simulink model "IndustrialMicrogrid"  (R2023a)
settings: Solver=FixedStepDiscrete  StartTime=0.0  StopTime=10  FixedStep=Ts  RelTol=1e-3
PostLoadFcn:
  | IndustrialMicrogridInputData
  | GfmGridFormingConverterInputParameters
model workspace (MAT data in the model file):
  caseNum = 2
undefined symbols (not defined in the file): base, BESS, DiscIntNeverNeededParam, grid, Grid, gridInverter, machine, microgrid, PV, PVInverter, PVTransformer, scrFactorRg, scrFactorXg, transformer, Ts
libraries: ee_lib x112, eeGeneralControl x104, nesl_utility_internal x64, simulink x56, nesl_utility x37, fl_lib x29, slpidlib x13, eeTransforms x11, eeTotalHarmonicDistorsion x8, eeRmsMeasurement x4, eeSinusoidalMeasurement x4, simulink_extras x2
(part 13 of 14)

== system IndustrialMicrogrid/MG1 Primary Substation/BESS and Controller/BESS/Grid-Forming Converter Control/Current Limiting/CurrentLimitingMethod/currentSaturation/If Action Subsystem ==
  Is : Inport
  Isd : Inport  Port=2
  Isq : Inport  Port=3
  Action Port : ActionPort
  Constant : Constant  Value=maxSatCurrentLimit
  Divide : Product  Inputs=*/
  Product : Product
  Product1 : Product
  Idmax : Outport
  Iqmax : Outport  Port=2
  wires:
  Constant/1 -> Divide/1
  Is/1 -> Divide/2
  Divide/1 -> Product1/2, Product/1
  Isd/1 -> Product1/1
  Isq/1 -> Product/2
  Product1/1 -> Idmax/1
  Product/1 -> Iqmax/1

== system IndustrialMicrogrid/MG1 Primary Substation/BESS and Controller/BESS/Grid-Forming Converter Control/Current Limiting/CurrentLimitingMethod/currentSaturation/If Action Subsystem1 ==
  Action Port : ActionPort
  Constant3 : Constant  Value=0
  Constant4 : Constant  Value=0
  Idmax : Outport
  Iqmax : Outport  Port=2
  wires:
  Constant4/1 -> Iqmax/1
  Constant3/1 -> Idmax/1

== system IndustrialMicrogrid/MG1 Primary Substation/BESS and Controller/BESS/Grid-Forming Converter Control/Grid Voltage Reactive Power Support/Modifying Reactive Power Reference/Changing the Power Reference/ActivePowerReference ==
  note: Ensure Pref sign is maintained
  Id : Inport
  Vd : Inport  Port=2
  Pref : Inport  Port=3
  Abs1 : Abs  SaturateOnIntegerOverflow=off
  Abs2 : Abs  SaturateOnIntegerOverflow=off
  Min : MinMax  Inputs=2
  Product : Product
  Product2 : Product
  Saturation : Saturate  UpperLimit=1  LowerLimit=-1
  Sign : Signum
  PrefNew : Outport
  wires:
  Pref/1 -> Abs1/1, Sign/1
  Id/1 -> Product/1
  Sign/1 -> Product2/2
  Abs1/1 -> Min/2
  Product/1 -> Abs2/1
  Min/1 -> Product2/1
  Product2/1 -> Saturation/1
  Abs2/1 -> Min/1
  Vd/1 -> Product/2
  Saturation/1 -> PrefNew/1

== system IndustrialMicrogrid/MG1 Primary Substation/BESS and Controller/BESS/Grid-Forming Converter Control/Grid Voltage Reactive Power Support/Modifying Reactive Power Reference/Changing the Power Reference/EstimateIdForGivenIq ==
  Iq : Inport
  Add Constant1 : Bias  Bias=1*1  SaturateOnIntegerOverflow=off
  Gain : Gain  Gain=-1
  Gain3 : Gain  Gain=0.9
  Sqrt : Sqrt
  Square : Math  Operator=square
  Id : Outport
  wires:
  Square/1 -> Gain/1
  Gain3/1 -> Id/1
  Gain/1 -> Add Constant1/1
  Sqrt/1 -> Gain3/1
  Add Constant1/1 -> Sqrt/1
  Iq/1 -> Square/1

== system IndustrialMicrogrid/MG1 Primary Substation/BESS and Controller/BESS/Grid-Forming Converter Control/Grid Voltage Reactive Power Support/Modifying Reactive Power Reference/Changing the Power Reference/EstimateIqForReactivePower ==
  note: Computing minimum reactive power as per GC0137
  Vmin : Inport
  Vd : Inport  Port=2
  Vs : Inport  Port=3
  Abs : Abs  SaturateOnIntegerOverflow=off
  Add : Sum
  Add Constant : Bias  Bias=1  SaturateOnIntegerOverflow=off
  GC0137 line slope : Gain  Gain=-1.4578
  Gain4 : Gain  Gain=1.5
  Saturation : Saturate  UpperLimit=1  LowerLimit=0
  Saturation1 : Saturate  UpperLimit=1  LowerLimit=-1
  Subtract : Sum  Inputs=+-
  Iq : Outport
  wires:
  Abs/1 -> GC0137 line slope/1
  GC0137 line slope/1 -> Add Constant/1
  Subtract/1 -> Gain4/1
  Saturation1/1 -> Add/1
  Gain4/1 -> Saturation1/1
  Vmin/1 -> Subtract/1
  Vs/1 -> Abs/1
  Vd/1 -> Subtract/2
  Add/1 -> Saturation/1
  Saturation/1 -> Iq/1
  Add Constant/1 -> Add/2

== system IndustrialMicrogrid/MG1 Primary Substation/BESS and Controller/BESS/Grid-Forming Converter Control/Grid Voltage Reactive Power Support/Modifying Reactive Power Reference/Changing the Power Reference/ReactivePowerReference ==
  Vd : Inport
  Iq : Inport  Port=2
  Compute Power : Product
  Constant : Constant  Value=0.3
  Gain2 : Gain  Gain=1.05
  Switch : Switch  Criteria=u2 > Threshold  Threshold=0.3  SaturateOnIntegerOverflow=off  InputSameDT=off
  QrefNew : Outport
  wires:
  Compute Power/1 -> QrefNew/1
  Gain2/1 -> Compute Power/2
  Constant/1 -> Switch/3
  Iq/1 -> Gain2/1
  Vd/1 -> Switch/2, Switch/1
  Switch/1 -> Compute Power/1

== system IndustrialMicrogrid/MG1 Primary Substation/BESS and Controller/BESS/Grid-Forming Converter Control/Measurement/Frequency Measurement/Frequency Measurement/If Action Subsystem ==
  V : Inport
  Time : Inport  Port=2
  Action Port : ActionPort  ActionPortLabel=if(u1 > 0.9)
  Constant1 : Constant  Value=initialFrequency
  Delay : Delay  DelayLength=1
  Delay1 : Delay  DelayLength=1
  Frequency estimation : Subsystem  TreatAsAtomicUnit=on
  Hit Crossing : HitCross
  Second-Order Filter : eeGeneralControl/Second-Order Filter  Commented=through  FilterType=Low-pass  fn=initialFrequency  Zeta=1  Ts=sampleTime  A0=0  Ph0=0  f0=0  b0=0
      settings: LibrarySourceBlock=ee_sl_lib/General Control/Second-Order Filter
  Switch : Switch  Criteria=u2 > Threshold  Threshold=1  SaturateOnIntegerOverflow=off  InputSameDT=off
  Freq : Outport
  wires:
  Second-Order Filter/1 -> Delay/1, Frequency estimation/1(sk), Hit Crossing/1
  Delay1/1 -> Frequency estimation/4(k-1)
  Hit Crossing/1 -> Frequency estimation/Trigger
  Delay/1 -> Frequency estimation/2(sk-1)
  V/1 -> Second-Order Filter/1
  Time/1 -> Switch/2, Delay1/1, Frequency estimation/3(k)
  Frequency estimation/1(f) -> Switch/1
  Constant1/1 -> Switch/3
  Switch/1 -> Freq/1

== system IndustrialMicrogrid/MG1 Primary Substation/BESS and Controller/BESS/Grid-Forming Converter Control/Measurement/Frequency Measurement/Frequency Measurement/If Action Subsystem1 ==
  Action Port : ActionPort  ActionPortLabel=else
  Constant1 : Constant  Value=initialFrequency
  Out1 : Outport
  wires:
  Constant1/1 -> Out1/1

== system IndustrialMicrogrid/MG1 Primary Substation/BESS and Controller/BESS/Grid-Forming Converter Control/Measurement/Frequency Measurement/Frequency Measurement/Postive Sequence ==
  abc : Inport
  Complex to Real-Imag : ComplexToRealImag
  Demux : Demux  Outputs=3
  Symmetrical-Components Transform : eeTransforms/Symmetrical-Components Transform  PowerInvariant=off
      settings: LibrarySourceBlock=|
      | ee_sl_lib/Mathematical
      | Transforms/Symmetrical-Components
      | Transform
  Terminator : Terminator
  Terminator1 : Terminator
  Terminator2 : Terminator
  Transpose : Math  Operator=transpose
  posSeq : Outport
  wires:
  Transpose/1 -> Symmetrical-Components Transform/1
  Symmetrical-Components Transform/1 -> Demux/1
  Complex to Real-Imag/1 -> posSeq/1
  Demux/1 -> Complex to Real-Imag/1
  abc/1 -> Transpose/1
  Complex to Real-Imag/2 -> Terminator/1
  Demux/2 -> Terminator1/1
  Demux/3 -> Terminator2/1

== system IndustrialMicrogrid/MG1 Primary Substation/BESS and Controller/BESS/Grid-Forming Converter Control/Power Control/ActivePowerControl/vsmControl/Damping Frequency ==
  fref : Inport
  ConstantFreqReference : Subsystem  VariantControl=constFreq
  WithFrequencyMeasurement : Subsystem  VariantControl=freqMeas
  fmeas : Outport

== system IndustrialMicrogrid/MG1 Primary Substation/BESS and Controller/BESS/Grid-Forming Converter Control/Power Control/ActivePowerControl/vsmControl/Power Reference Selection ==
  cntrlflag : Inport
  Pref : Inport  Port=2
  fref : Inport  Port=3
  Wsm : Inport  Port=4
  If : If
  If Action Subsystem : Subsystem  TreatAsAtomicUnit=on
  If Action Subsystem1 : Subsystem  TreatAsAtomicUnit=on
  Merge : Merge
  power : Outport
  wires:
  If Action Subsystem1/1(Power) -> Merge/2
  If/1 -> If Action Subsystem/Action
  Pref/1 -> If Action Subsystem/1(Pref)
  [Wsm] -> If Action Subsystem1/2(Wsm)
  fref/1 -> If Action Subsystem1/1(fref)
  [Wsm] -> If Action Subsystem/2(Wsm)
  If Action Subsystem/1(Power) -> Merge/1
  If/2 -> If Action Subsystem1/Action
  cntrlflag/1 -> If/1
  Merge/1 -> power/1
  Wsm/1 -> [Wsm]

== system IndustrialMicrogrid/MG1 Primary Substation/BESS and Controller/BESS/Grid-Forming Converter Control/Power Control/ReactiveControl/Voltage  Reference Selection/If Action Subsystem ==
  note: Vs-delV
  Qref : Inport
  Qmeas : Inport  Port=2
  Action Port : ActionPort  ActionPortLabel=if(u1 > 0)
  Constant : Constant  Value=voltreference
  Gain : Gain  Gain=QVoltDroop
  Low-Pass Filter (Discrete or Continuous) : eeGeneralControl/Low-Pass Filter (Discrete or Continuous)  K=1  T=QVoltFilterTC  B=inf  A=-inf  init_option=Specify as parameter  x0=0  Ts=activePowerSampleTime
  Product1 : Product
  Sum : Sum  Inputs=|+-
  Sum1 : Sum  Inputs=|++
  Vd : Outport
  wires:
  Constant/1 -> Product1/2, Sum1/2
  Qmeas/1 -> Low-Pass Filter (Discrete or Continuous)/1
  Gain/1 -> Sum1/1
  Qref/1 -> Sum/1
  Low-Pass Filter (Discrete or Continuous)/1 -> Sum/2
  Sum/1 -> Gain/1
  Sum1/1 -> Product1/1
  Product1/1 -> Vd/1  "V"

== system IndustrialMicrogrid/MG1 Primary Substation/BESS and Controller/BESS/Grid-Forming Converter Control/Power Control/ReactiveControl/Voltage  Reference Selection/If Action Subsystem1 ==
  note: Vs-delV
  Vref : Inport
  Vmeas : Inport  Port=2
  Action Port : ActionPort  ActionPortLabel=else
  Constant : Constant  Value=voltreference
  Gain : Gain  Gain=1/QVoltDroop
  Low-Pass Filter (Discrete or Continuous) : eeGeneralControl/Low-Pass Filter (Discrete or Continuous)  K=1  T=QVoltFilterTC  B=inf  A=-inf  init_option=Specify as parameter  x0=0  Ts=activePowerSampleTime
  Product1 : Product
  Scope : Scope
  Scope1 : Scope
  Scope2 : Scope
  Sum : Sum  Inputs=|+-
  Sum1 : Sum  Inputs=|++
  Voltage : Outport
  wires:
  Vref/1 -> Voltage/1, Product1/1, Sum/1
  Gain/1 -> Sum1/1
  Vmeas/1 -> Low-Pass Filter (Discrete or Continuous)/1
  Constant/1 -> Sum1/2
  Low-Pass Filter (Discrete or Continuous)/1 -> Sum/2, Scope1/1
  Sum/1 -> Scope2/1, Gain/1
  Product1/1 -> Scope/1  "V"
  Sum1/1 -> Product1/2

== system IndustrialMicrogrid/MG2 Primary Substation/BESS and Controller 2/BESS/Grid-Forming Converter Control/Current Limiting/CurrentLimitingMethod/currentLimitAndVirtual/Current Saturation ==
  note: Vs-delV
  Id : Inport
  Iq : Inport  Port=2
  Imaxsat : Inport  Port=3
  Enable : EnablePort
  Compare : Subsystem
  Constant1 : Constant  Value=0
  Constant2 : Constant  Value=0
  If : If
  If Action Subsystem : Subsystem  TreatAsAtomicUnit=on
  If Action Subsystem1 : Subsystem  TreatAsAtomicUnit=on
  Math Function : Math  Operator=hypot
  Merge : Merge
  Merge1 : Merge
  Subtract : Sum  Inputs=+-
  delVd : Outport
  delVq : Outport  Port=2
  idmax : Outport  Port=3
  iqmax : Outport  Port=4
  wires:
  Iq/1 -> [Isq], Math Function/2
  If/1 -> If Action Subsystem/Action
  If Action Subsystem1/1(Idmax) -> Merge/2
  Constant2/1 -> delVq/1
  Math Function/1 -> [Is], Subtract/2
  If/2 -> If Action Subsystem1/Action
  If Action Subsystem/2(Iqmax) -> Merge1/1
  Subtract/1 -> Compare/1(u)
  Compare/1(Out1) -> If/1
  If Action Subsystem/1(Idmax) -> Merge/1
  [Is] -> If Action Subsystem/1(Is)
  Id/1 -> [Isd], Math Function/1
  If Action Subsystem1/2(Iqmax) -> Merge1/2
  Merge/1 -> idmax/1
  [Isd] -> If Action Subsystem/2(Isd)
  Constant1/1 -> delVd/1
  [Isq] -> If Action Subsystem/3(Isq)
  Merge1/1 -> iqmax/1
  Imaxsat/1 -> [Imax], Subtract/1
  [Imax] -> If Action Subsystem/4(maxI)

== system IndustrialMicrogrid/MG2 Primary Substation/BESS and Controller 2/BESS/Grid-Forming Converter Control/Current Limiting/CurrentLimitingMethod/currentLimitAndVirtual/No Fault Ride Through ==
  Id : Inport
  Iq : Inport  Port=2
  Enable : EnablePort
  Constant{1..4} (4 alike) : Constant  Value=0
  Terminator : Terminator
  Terminator1 : Terminator
  delVd : Outport
  delVq : Outport  Port=2
  idmax : Outport  Port=3
  iqmax : Outport  Port=4
  wires:
  Constant3/1 -> iqmax/1
  Constant2/1 -> idmax/1
  Constant1/1 -> delVd/1
  Constant4/1 -> delVq/1
  Id/1 -> Terminator/1
  Iq/1 -> Terminator1/1

== system IndustrialMicrogrid/MG2 Primary Substation/BESS and Controller 2/BESS/Grid-Forming Converter Control/Current Limiting/CurrentLimitingMethod/currentLimitAndVirtual/VI ==
  note: Resistance coefficient
  note: X/R ratio
  Id : Inport
  Iq : Inport  Port=2
  Imax : Inport  Port=3
  Enable : EnablePort
  Constant1 : Constant  Value=0
  Constant2 : Constant  Value=0
  Constant3 : Constant  Value=0
  Gain : Gain  Gain=ctLimitVirtualImp
  Gain1 : Gain  Gain=ctLimitXbyR
  Low-Pass Filter : eeGeneralControl/Low-Pass Filter (Discrete or Continuous)  K=1  T=currentVITimeConst  B=inf  A=-inf  init_option=Inherited from block input  x0=0  Ts=-1
  Math Function : Math  Operator=hypot
  Product{,1..3} (4 alike) : Product
  Relay1 : Relay  OnSwitchValue=0.01  OffSwitchValue=-0.1
  Saturation : Saturate  UpperLimit=1  LowerLimit=-1
  Saturation1 : Saturate  UpperLimit=1  LowerLimit=-1
  Sum : Sum  Inputs=|+-
  Sum1 : Sum  Inputs=|+-
  Sum2 : Sum  Inputs=++|
  Switch : Switch  Criteria=u2 > Threshold  SaturateOnIntegerOverflow=off  InputSameDT=off
  delVd : Outport
  delVq : Outport  Port=2
  idmax : Outport  Port=3
  iqmax : Outport  Port=4
  wires:
  Gain1/1 -> Product1/2, Product2/1
  Product3/1 -> Sum2/2
  Id/1 -> Math Function/1, [Igd]
  Sum2/1 -> Saturation1/1
  Sum/1 -> Gain/1, Relay1/1
  Sum1/1 -> Saturation/1
  Product/1 -> Sum1/1
  [Igq] -> Product3/1, Product2/2
  Iq/1 -> [Igq], Math Function/2
  Math Function/1 -> Low-Pass Filter/1  "Is"
  Switch/1 -> Product3/2, Product/1, Gain1/1
  [Igd] -> Product1/1, Product/2
  Saturation1/1 -> delVq/1
  Product1/1 -> Sum2/1
  Product2/1 -> Sum1/2
  Gain/1 -> Switch/1
  Constant1/1 -> Switch/3
  Saturation/1 -> delVd/1
  Constant3/1 -> iqmax/1
  Constant2/1 -> idmax/1
  Relay1/1 -> Switch/2
  Low-Pass Filter/1 -> Sum/1
  Imax/1 -> Sum/2  "IsMaximum"

== system IndustrialMicrogrid/MG2 Primary Substation/BESS and Controller 2/BESS/Grid-Forming Converter Control/Current Limiting/CurrentLimitingMethod/currentSaturation/Compare ==
  u : Inport
  AND : Logic  IconShape=distinctive  AllPortsSameDT=off  OutDataTypeStr=boolean
  Compare To Constant : simulink/Logic and Bit Operations/Compare To Constant  relop=>  const=ctLimitDelayTime  OutDataTypeStr=boolean
  Compare To Zero : simulink/Logic and Bit Operations/Compare To Zero  relop=<=  OutDataTypeStr=boolean
  Data Type Conversion : DataTypeConversion  SaturateOnIntegerOverflow=off  RndMeth=Floor
  Data Type Conversion1 : DataTypeConversion  SaturateOnIntegerOverflow=off  RndMeth=Floor
  Discrete-Time Integrator : DiscreteIntegrator  IntegratorMethod=Integration: Backward Euler  ExternalReset=level  SampleTime=currentControlTs  LimitOutput=on  UpperSaturationLimit=ctLimitDelayTime*2  LowerSaturationLimit=0  ICPrevOutput=DiscIntNeverNeededParam  ICPrevScaledInput=DiscIntNeverNeededParam
  Out1 : Outport
  wires:
  AND/1 -> Data Type Conversion/1
  Compare To Zero/1 -> Data Type Conversion1/1
  Compare To Constant/1 -> AND/2
  u/1 -> Compare To Zero/1
  Discrete-Time Integrator/1 -> Compare To Constant/1
  Data Type Conversion/1 -> Out1/1
  Data Type Conversion1/1 -> Discrete-Time Integrator/2, Discrete-Time Integrator/1, AND/1

== system IndustrialMicrogrid/MG2 Primary Substation/BESS and Controller 2/BESS/Grid-Forming Converter Control/Current Limiting/CurrentLimitingMethod/currentSaturation/If Action Subsystem ==
  Is : Inport
  Isd : Inport  Port=2
  Isq : Inport  Port=3
  Action Port : ActionPort
  Constant : Constant  Value=maxSatCurrentLimit
  Divide : Product  Inputs=*/
  Product : Product
  Product1 : Product
  Idmax : Outport
  Iqmax : Outport  Port=2
  wires:
  Constant/1 -> Divide/1
  Is/1 -> Divide/2
  Divide/1 -> Product1/2, Product/1
  Isd/1 -> Product1/1
  Isq/1 -> Product/2
  Product1/1 -> Idmax/1
  Product/1 -> Iqmax/1

== system IndustrialMicrogrid/MG2 Primary Substation/BESS and Controller 2/BESS/Grid-Forming Converter Control/Current Limiting/CurrentLimitingMethod/currentSaturation/If Action Subsystem1 ==
  Action Port : ActionPort
  Constant3 : Constant  Value=0
  Constant4 : Constant  Value=0
  Idmax : Outport
  Iqmax : Outport  Port=2
  wires:
  Constant4/1 -> Iqmax/1
  Constant3/1 -> Idmax/1

== system IndustrialMicrogrid/MG2 Primary Substation/BESS and Controller 2/BESS/Grid-Forming Converter Control/Grid Voltage Reactive Power Support/Modifying Reactive Power Reference/Changing the Power Reference/ActivePowerReference ==
  note: Ensure Pref sign is maintained
  Id : Inport
  Vd : Inport  Port=2
  Pref : Inport  Port=3
  Abs1 : Abs  SaturateOnIntegerOverflow=off
  Abs2 : Abs  SaturateOnIntegerOverflow=off
  Min : MinMax  Inputs=2
  Product : Product
  Product2 : Product
  Saturation : Saturate  UpperLimit=1  LowerLimit=-1
  Sign : Signum
  PrefNew : Outport
  wires:
  Pref/1 -> Abs1/1, Sign/1
  Id/1 -> Product/1
  Sign/1 -> Product2/2
  Abs1/1 -> Min/2
  Product/1 -> Abs2/1
  Min/1 -> Product2/1
  Product2/1 -> Saturation/1
  Abs2/1 -> Min/1
  Vd/1 -> Product/2
  Saturation/1 -> PrefNew/1

== system IndustrialMicrogrid/MG2 Primary Substation/BESS and Controller 2/BESS/Grid-Forming Converter Control/Grid Voltage Reactive Power Support/Modifying Reactive Power Reference/Changing the Power Reference/EstimateIdForGivenIq ==
  Iq : Inport
  Add Constant1 : Bias  Bias=1*1  SaturateOnIntegerOverflow=off
  Gain : Gain  Gain=-1
  Gain3 : Gain  Gain=0.9
  Sqrt : Sqrt
  Square : Math  Operator=square
  Id : Outport
  wires:
  Square/1 -> Gain/1
  Gain3/1 -> Id/1
  Gain/1 -> Add Constant1/1
  Sqrt/1 -> Gain3/1
  Add Constant1/1 -> Sqrt/1
  Iq/1 -> Square/1

== system IndustrialMicrogrid/MG2 Primary Substation/BESS and Controller 2/BESS/Grid-Forming Converter Control/Grid Voltage Reactive Power Support/Modifying Reactive Power Reference/Changing the Power Reference/EstimateIqForReactivePower ==
  note: Computing minimum reactive power as per GC0137
  Vmin : Inport
  Vd : Inport  Port=2
  Vs : Inport  Port=3
  Abs : Abs  SaturateOnIntegerOverflow=off
  Add : Sum
  Add Constant : Bias  Bias=1  SaturateOnIntegerOverflow=off
  GC0137 line slope : Gain  Gain=-1.4578
  Gain4 : Gain  Gain=1.5
  Saturation : Saturate  UpperLimit=1  LowerLimit=0
  Saturation1 : Saturate  UpperLimit=1  LowerLimit=-1
  Subtract : Sum  Inputs=+-
  Iq : Outport
  wires:
  Abs/1 -> GC0137 line slope/1
  GC0137 line slope/1 -> Add Constant/1
  Subtract/1 -> Gain4/1
  Saturation1/1 -> Add/1
  Gain4/1 -> Saturation1/1
  Vmin/1 -> Subtract/1
  Vs/1 -> Abs/1
  Vd/1 -> Subtract/2
  Add/1 -> Saturation/1
  Saturation/1 -> Iq/1
  Add Constant/1 -> Add/2

== system IndustrialMicrogrid/MG2 Primary Substation/BESS and Controller 2/BESS/Grid-Forming Converter Control/Grid Voltage Reactive Power Support/Modifying Reactive Power Reference/Changing the Power Reference/ReactivePowerReference ==
  Vd : Inport
  Iq : Inport  Port=2
  Compute Power : Product
  Constant : Constant  Value=0.3
  Gain2 : Gain  Gain=1.05
  Switch : Switch  Criteria=u2 > Threshold  Threshold=0.3  SaturateOnIntegerOverflow=off  InputSameDT=off
  QrefNew : Outport
  wires:
  Compute Power/1 -> QrefNew/1
  Gain2/1 -> Compute Power/2
  Constant/1 -> Switch/3
  Iq/1 -> Gain2/1
  Vd/1 -> Switch/2, Switch/1
  Switch/1 -> Compute Power/1

== system IndustrialMicrogrid/MG2 Primary Substation/BESS and Controller 2/BESS/Grid-Forming Converter Control/Measurement/Frequency Measurement/Frequency Measurement/If Action Subsystem ==
  V : Inport
  Time : Inport  Port=2
  Action Port : ActionPort  ActionPortLabel=if(u1 > 0.9)
  Constant1 : Constant  Value=initialFrequency
  Delay : Delay  DelayLength=1
  Delay1 : Delay  DelayLength=1
  Frequency estimation : Subsystem  TreatAsAtomicUnit=on
  Hit Crossing : HitCross
  Second-Order Filter : eeGeneralControl/Second-Order Filter  Commented=through  FilterType=Low-pass  fn=initialFrequency  Zeta=1  Ts=sampleTime  A0=0  Ph0=0  f0=0  b0=0
      settings: LibrarySourceBlock=ee_sl_lib/General Control/Second-Order Filter
  Switch : Switch  Criteria=u2 > Threshold  Threshold=1  SaturateOnIntegerOverflow=off  InputSameDT=off
  Freq : Outport
  wires:
  Second-Order Filter/1 -> Delay/1, Frequency estimation/1(sk), Hit Crossing/1
  Delay1/1 -> Frequency estimation/4(k-1)
  Hit Crossing/1 -> Frequency estimation/Trigger
  Delay/1 -> Frequency estimation/2(sk-1)
  V/1 -> Second-Order Filter/1
  Time/1 -> Switch/2, Delay1/1, Frequency estimation/3(k)
  Frequency estimation/1(f) -> Switch/1
  Constant1/1 -> Switch/3
  Switch/1 -> Freq/1

== system IndustrialMicrogrid/MG2 Primary Substation/BESS and Controller 2/BESS/Grid-Forming Converter Control/Measurement/Frequency Measurement/Frequency Measurement/If Action Subsystem1 ==
  Action Port : ActionPort  ActionPortLabel=else
  Constant1 : Constant  Value=initialFrequency
  Out1 : Outport
  wires:
  Constant1/1 -> Out1/1

== system IndustrialMicrogrid/MG2 Primary Substation/BESS and Controller 2/BESS/Grid-Forming Converter Control/Measurement/Frequency Measurement/Frequency Measurement/Postive Sequence ==
  abc : Inport
  Complex to Real-Imag : ComplexToRealImag
  Demux : Demux  Outputs=3
  Symmetrical-Components Transform : eeTransforms/Symmetrical-Components Transform  PowerInvariant=off
      settings: LibrarySourceBlock=|
      | ee_sl_lib/Mathematical
      | Transforms/Symmetrical-Components
      | Transform
  Terminator : Terminator
  Terminator1 : Terminator
  Terminator2 : Terminator
  Transpose : Math  Operator=transpose
  posSeq : Outport
  wires:
  Transpose/1 -> Symmetrical-Components Transform/1
  Symmetrical-Components Transform/1 -> Demux/1
  Complex to Real-Imag/1 -> posSeq/1
  Demux/1 -> Complex to Real-Imag/1
  abc/1 -> Transpose/1
  Complex to Real-Imag/2 -> Terminator/1
  Demux/2 -> Terminator1/1
  Demux/3 -> Terminator2/1

== system IndustrialMicrogrid/MG2 Primary Substation/BESS and Controller 2/BESS/Grid-Forming Converter Control/Power Control/ActivePowerControl/vsmControl/Damping Frequency ==
  fref : Inport
  ConstantFreqReference : Subsystem  VariantControl=constFreq
  WithFrequencyMeasurement : Subsystem  VariantControl=freqMeas
  fmeas : Outport

== system IndustrialMicrogrid/MG2 Primary Substation/BESS and Controller 2/BESS/Grid-Forming Converter Control/Power Control/ActivePowerControl/vsmControl/Power Reference Selection ==
  cntrlflag : Inport
  Pref : Inport  Port=2
  fref : Inport  Port=3
  Wsm : Inport  Port=4
  If : If
  If Action Subsystem : Subsystem  TreatAsAtomicUnit=on
  If Action Subsystem1 : Subsystem  TreatAsAtomicUnit=on
  Merge : Merge
  power : Outport
  wires:
  If Action Subsystem1/1(Power) -> Merge/2
  If/1 -> If Action Subsystem/Action
  Pref/1 -> If Action Subsystem/1(Pref)
  [Wsm] -> If Action Subsystem1/2(Wsm)
  fref/1 -> If Action Subsystem1/1(fref)
  [Wsm] -> If Action Subsystem/2(Wsm)
  If Action Subsystem/1(Power) -> Merge/1
  If/2 -> If Action Subsystem1/Action
  cntrlflag/1 -> If/1
  Merge/1 -> power/1
  Wsm/1 -> [Wsm]

== system IndustrialMicrogrid/MG2 Primary Substation/BESS and Controller 2/BESS/Grid-Forming Converter Control/Power Control/ReactiveControl/Voltage  Reference Selection/If Action Subsystem ==
  note: Vs-delV
  Qref : Inport
  Qmeas : Inport  Port=2
  Action Port : ActionPort  ActionPortLabel=if(u1 > 0)
  Constant : Constant  Value=voltreference
  Gain : Gain  Gain=QVoltDroop
  Low-Pass Filter (Discrete or Continuous) : eeGeneralControl/Low-Pass Filter (Discrete or Continuous)  K=1  T=QVoltFilterTC  B=inf  A=-inf  init_option=Specify as parameter  x0=0  Ts=activePowerSampleTime
  Product1 : Product
  Sum : Sum  Inputs=|+-
  Sum1 : Sum  Inputs=|++
  Vd : Outport
  wires:
  Constant/1 -> Product1/2, Sum1/2
  Qmeas/1 -> Low-Pass Filter (Discrete or Continuous)/1
  Gain/1 -> Sum1/1
  Qref/1 -> Sum/1
  Low-Pass Filter (Discrete or Continuous)/1 -> Sum/2
  Sum/1 -> Gain/1
  Sum1/1 -> Product1/1
  Product1/1 -> Vd/1  "V"

== system IndustrialMicrogrid/MG2 Primary Substation/BESS and Controller 2/BESS/Grid-Forming Converter Control/Power Control/ReactiveControl/Voltage  Reference Selection/If Action Subsystem1 ==
  note: Vs-delV
  Vref : Inport
  Vmeas : Inport  Port=2
  Action Port : ActionPort  ActionPortLabel=else
  Constant : Constant  Value=voltreference
  Gain : Gain  Gain=1/QVoltDroop
  Low-Pass Filter (Discrete or Continuous) : eeGeneralControl/Low-Pass Filter (Discrete or Continuous)  K=1  T=QVoltFilterTC  B=inf  A=-inf  init_option=Specify as parameter  x0=0  Ts=activePowerSampleTime
  Product1 : Product
  Scope : Scope
  Scope1 : Scope
  Scope2 : Scope
  Sum : Sum  Inputs=|+-
  Sum1 : Sum  Inputs=|++
  Voltage : Outport
  wires:
  Vref/1 -> Voltage/1, Product1/1, Sum/1
  Gain/1 -> Sum1/1
  Vmeas/1 -> Low-Pass Filter (Discrete or Continuous)/1
  Constant/1 -> Sum1/2
  Low-Pass Filter (Discrete or Continuous)/1 -> Sum/2, Scope1/1
  Sum/1 -> Scope2/1, Gain/1
  Product1/1 -> Scope/1  "V"
  Sum1/1 -> Product1/2

== system IndustrialMicrogrid/Operator Room/OperatorControlRoom/MG1 Controller : Commands and Measurements/Microgrid Controller 1 : Commands and Measurements/Measurements and visualizations /BESS, PV and Load Measurements/BESS and PV Measurements/Inverter Active & Reactive Power  ==
  Vabc : Inport
  Iabc : Inport  Port=2
  Demux : Demux  Outputs=3
  Gain : Gain  Gain=1/sqrt(3)
  Low-Pass Filter (Discrete or Continuous) : eeGeneralControl/Low-Pass Filter (Discrete or Continuous)  K=1  T=0.02  B=inf  A=-inf  init_option=Inherited from block input  x0=0  Ts=-1
  Low-Pass Filter (Discrete or Continuous)1 : eeGeneralControl/Low-Pass Filter (Discrete or Continuous)  K=1  T=0.02  B=inf  A=-inf  init_option=Inherited from block input  x0=0  Ts=-1
  Minus : Sum  Inputs=+-
  Minus1 : Sum  Inputs=+-
  Minus2 : Sum  Inputs=+-
  Mux : Mux  Inputs=3
  Product : Product
  Product1 : Product
  Sum of Elements : Sum  Inputs=+
  Sum of Elements1 : Sum  Inputs=+
  gain : Gain  Gain=2/3
  gain1 : Gain  Gain=2/3
  P : Outport  VectorParamsAs1DForOutWhenUnconnected=off
  Q : Outport  Port=2  VectorParamsAs1DForOutWhenUnconnected=off
  wires:
  Minus/1 -> Mux/3
  Minus2/1 -> Mux/2
  Minus1/1 -> Mux/1
  Gain/1 -> Low-Pass Filter (Discrete or Continuous)1/1
  Sum of Elements1/1 -> Gain/1
  Product1/1 -> Sum of Elements1/1
  Mux/1 -> Product1/2
  Demux/3 -> Minus1/2, Minus2/1
  Demux/2 -> Minus/2, Minus1/1
  Demux/1 -> Minus/1, Minus2/2
  Sum of Elements/1 -> Low-Pass Filter (Discrete or Continuous)/1
  Product/1 -> Sum of Elements/1
  Iabc/1 -> Product/2, Product1/1
  Vabc/1 -> Product/1, Demux/1
  Low-Pass Filter (Discrete or Continuous)/1 -> gain/1
  Low-Pass Filter (Discrete or Continuous)1/1 -> gain1/1
  gain/1 -> P/1  "BESS Active Power(pu)"
  gain1/1 -> Q/1  "BESS Reactive Power(pu)"

== system IndustrialMicrogrid/Operator Room/OperatorControlRoom/MG1 Controller : Commands and Measurements/Microgrid Controller 1 : Commands and Measurements/Measurements and visualizations /Resynchronization and Planned Islanding/Planned Islanding/Grid Active & Reactive Power  ==
  Vabc : Inport
  Iabc : Inport  Port=2
  Demux : Demux  Outputs=3
  Gain : Gain  Gain=1/sqrt(3)
  Low-Pass Filter (Discrete or Continuous) : eeGeneralControl/Low-Pass Filter (Discrete or Continuous)  K=1  T=0.02  B=inf  A=-inf  init_option=Inherited from block input  x0=0  Ts=-1
  Low-Pass Filter (Discrete or Continuous)1 : eeGeneralControl/Low-Pass Filter (Discrete or Continuous)  K=1  T=0.02  B=inf  A=-inf  init_option=Inherited from block input  x0=0  Ts=-1
  Minus : Sum  Inputs=+-
  Minus1 : Sum  Inputs=+-
  Minus2 : Sum  Inputs=+-
  Mux : Mux  Inputs=3
  Product : Product
  Product1 : Product
  Sum of Elements : Sum  Inputs=+
  Sum of Elements1 : Sum  Inputs=+
  gain : Gain  Gain=2/3
  gain1 : Gain  Gain=2/3
  P : Outport  VectorParamsAs1DForOutWhenUnconnected=off
  Q : Outport  Port=2  VectorParamsAs1DForOutWhenUnconnected=off
  wires:
  Minus/1 -> Mux/3
  Minus2/1 -> Mux/2
  Minus1/1 -> Mux/1
  Gain/1 -> Low-Pass Filter (Discrete or Continuous)1/1
  Sum of Elements1/1 -> Gain/1
  Product1/1 -> Sum of Elements1/1
  Mux/1 -> Product1/2
  Demux/3 -> Minus1/2, Minus2/1
  Demux/2 -> Minus/2, Minus1/1
  Demux/1 -> Minus/1, Minus2/2
  Sum of Elements/1 -> Low-Pass Filter (Discrete or Continuous)/1
  Product/1 -> Sum of Elements/1
  Iabc/1 -> Product/2, Product1/1
  Vabc/1 -> Product/1, Demux/1
  Low-Pass Filter (Discrete or Continuous)/1 -> gain/1
  Low-Pass Filter (Discrete or Continuous)1/1 -> gain1/1
  gain/1 -> P/1  "BESS Active Power(pu)"
  gain1/1 -> Q/1  "BESS Reactive Power(pu)"

== system IndustrialMicrogrid/Operator Room/OperatorControlRoom/MG1 Controller : Commands and Measurements/Microgrid Controller 1 : Commands and Measurements/Measurements and visualizations /Resynchronization and Planned Islanding/Resync/Grid Active & Reactive Power  ==
  Vabc : Inport
  Iabc : Inport  Port=2
  Demux : Demux  Outputs=3
  Gain : Gain  Gain=1/sqrt(3)
  Low-Pass Filter (Discrete or Continuous) : eeGeneralControl/Low-Pass Filter (Discrete or Continuous)  K=1  T=0.02  B=inf  A=-inf  init_option=Inherited from block input  x0=0  Ts=-1
  Low-Pass Filter (Discrete or Continuous)1 : eeGeneralControl/Low-Pass Filter (Discrete or Continuous)  K=1  T=0.02  B=inf  A=-inf  init_option=Inherited from block input  x0=0  Ts=-1
  Minus : Sum  Inputs=+-
  Minus1 : Sum  Inputs=+-
  Minus2 : Sum  Inputs=+-
  Mux : Mux  Inputs=3
  Product : Product
  Product1 : Product
  Sum of Elements : Sum  Inputs=+
  Sum of Elements1 : Sum  Inputs=+
  gain : Gain  Gain=2/3
  gain1 : Gain  Gain=2/3
  P : Outport  VectorParamsAs1DForOutWhenUnconnected=off
  Q : Outport  Port=2  VectorParamsAs1DForOutWhenUnconnected=off
  wires:
  Minus/1 -> Mux/3
  Minus2/1 -> Mux/2
  Minus1/1 -> Mux/1
  Gain/1 -> Low-Pass Filter (Discrete or Continuous)1/1
  Sum of Elements1/1 -> Gain/1
  Product1/1 -> Sum of Elements1/1
  Mux/1 -> Product1/2
  Demux/3 -> Minus1/2, Minus2/1
  Demux/2 -> Minus/2, Minus1/1
  Demux/1 -> Minus/1, Minus2/2
  Sum of Elements/1 -> Low-Pass Filter (Discrete or Continuous)/1
  Product/1 -> Sum of Elements/1
  Iabc/1 -> Product/2, Product1/1
  Vabc/1 -> Product/1, Demux/1
  Low-Pass Filter (Discrete or Continuous)/1 -> gain/1
  Low-Pass Filter (Discrete or Continuous)1/1 -> gain1/1
  gain/1 -> P/1  "BESS Active Power(pu)"
  gain1/1 -> Q/1  "BESS Reactive Power(pu)"

== system IndustrialMicrogrid/Operator Room/OperatorControlRoom/MG2 Controller : Commands and Measurements/Microgrid Controller 2 : Commands and Measurements/Measurements and visualizations 1/BESS, PV and Load Measurements/BESS and PV Measurements/Inverter Active & Reactive Power  ==
  Vabc : Inport
  Iabc : Inport  Port=2
  Demux : Demux  Outputs=3
  Gain : Gain  Gain=1/sqrt(3)
  Low-Pass Filter (Discrete or Continuous) : eeGeneralControl/Low-Pass Filter (Discrete or Continuous)  K=1  T=0.02  B=inf  A=-inf  init_option=Inherited from block input  x0=0  Ts=-1
  Low-Pass Filter (Discrete or Continuous)1 : eeGeneralControl/Low-Pass Filter (Discrete or Continuous)  K=1  T=0.02  B=inf  A=-inf  init_option=Inherited from block input  x0=0  Ts=-1
  Minus : Sum  Inputs=+-
  Minus1 : Sum  Inputs=+-
  Minus2 : Sum  Inputs=+-
  Mux : Mux  Inputs=3
  Product : Product
  Product1 : Product
  Sum of Elements : Sum  Inputs=+
  Sum of Elements1 : Sum  Inputs=+
  gain : Gain  Gain=2/3
  gain1 : Gain  Gain=2/3
  P : Outport  VectorParamsAs1DForOutWhenUnconnected=off
  Q : Outport  Port=2  VectorParamsAs1DForOutWhenUnconnected=off
  wires:
  Minus/1 -> Mux/3
  Minus2/1 -> Mux/2
  Minus1/1 -> Mux/1
  Gain/1 -> Low-Pass Filter (Discrete or Continuous)1/1
  Sum of Elements1/1 -> Gain/1
  Product1/1 -> Sum of Elements1/1
  Mux/1 -> Product1/2
  Demux/3 -> Minus1/2, Minus2/1
  Demux/2 -> Minus/2, Minus1/1
  Demux/1 -> Minus/1, Minus2/2
  Sum of Elements/1 -> Low-Pass Filter (Discrete or Continuous)/1
  Product/1 -> Sum of Elements/1
  Iabc/1 -> Product/2, Product1/1
  Vabc/1 -> Product/1, Demux/1
  Low-Pass Filter (Discrete or Continuous)/1 -> gain/1
  Low-Pass Filter (Discrete or Continuous)1/1 -> gain1/1
  gain/1 -> P/1  "BESS Active Power(pu)"
  gain1/1 -> Q/1  "BESS Reactive Power(pu)"

== system IndustrialMicrogrid/Operator Room/OperatorControlRoom/MG2 Controller : Commands and Measurements/Microgrid Controller 2 : Commands and Measurements/Measurements and visualizations 1/Resynchronization and Planned Islanding/Planned Islanding/Grid Active & Reactive Power  ==
  Vabc : Inport
  Iabc : Inport  Port=2
  Demux : Demux  Outputs=3
  Gain : Gain  Gain=1/sqrt(3)
  Low-Pass Filter (Discrete or Continuous) : eeGeneralControl/Low-Pass Filter (Discrete or Continuous)  K=1  T=0.02  B=inf  A=-inf  init_option=Inherited from block input  x0=0  Ts=-1
  Low-Pass Filter (Discrete or Continuous)1 : eeGeneralControl/Low-Pass Filter (Discrete or Continuous)  K=1  T=0.02  B=inf  A=-inf  init_option=Inherited from block input  x0=0  Ts=-1
  Minus : Sum  Inputs=+-
  Minus1 : Sum  Inputs=+-
  Minus2 : Sum  Inputs=+-
  Mux : Mux  Inputs=3
  Product : Product
  Product1 : Product
  Sum of Elements : Sum  Inputs=+
  Sum of Elements1 : Sum  Inputs=+
  gain : Gain  Gain=2/3
  gain1 : Gain  Gain=2/3
  P : Outport  VectorParamsAs1DForOutWhenUnconnected=off
  Q : Outport  Port=2  VectorParamsAs1DForOutWhenUnconnected=off
  wires:
  gain1/1 -> Q/1  "BESS Reactive Power(pu)"
  gain/1 -> P/1  "BESS Active Power(pu)"
  Low-Pass Filter (Discrete or Continuous)1/1 -> gain1/1
  Low-Pass Filter (Discrete or Continuous)/1 -> gain/1
  Vabc/1 -> Demux/1, Product/1
  Iabc/1 -> Product1/1, Product/2
  Product/1 -> Sum of Elements/1
  Sum of Elements/1 -> Low-Pass Filter (Discrete or Continuous)/1
  Demux/1 -> Minus2/2, Minus/1
  Demux/2 -> Minus1/1, Minus/2
  Demux/3 -> Minus2/1, Minus1/2
  Mux/1 -> Product1/2
  Product1/1 -> Sum of Elements1/1
  Sum of Elements1/1 -> Gain/1
  Gain/1 -> Low-Pass Filter (Discrete or Continuous)1/1
  Minus1/1 -> Mux/1
  Minus2/1 -> Mux/2
  Minus/1 -> Mux/3

== system IndustrialMicrogrid/Operator Room/OperatorControlRoom/MG2 Controller : Commands and Measurements/Microgrid Controller 2 : Commands and Measurements/Measurements and visualizations 1/Resynchronization and Planned Islanding/Resync/Grid Active & Reactive Power  ==
  Vabc : Inport
  Iabc : Inport  Port=2
  Demux : Demux  Outputs=3
  Gain : Gain  Gain=1/sqrt(3)
  Low-Pass Filter (Discrete or Continuous) : eeGeneralControl/Low-Pass Filter (Discrete or Continuous)  K=1  T=0.02  B=inf  A=-inf  init_option=Inherited from block input  x0=0  Ts=-1
  Low-Pass Filter (Discrete or Continuous)1 : eeGeneralControl/Low-Pass Filter (Discrete or Continuous)  K=1  T=0.02  B=inf  A=-inf  init_option=Inherited from block input  x0=0  Ts=-1
  Minus : Sum  Inputs=+-
  Minus1 : Sum  Inputs=+-
  Minus2 : Sum  Inputs=+-
  Mux : Mux  Inputs=3
  Product : Product
  Product1 : Product
  Sum of Elements : Sum  Inputs=+
  Sum of Elements1 : Sum  Inputs=+
  gain : Gain  Gain=2/3
  gain1 : Gain  Gain=2/3
  P : Outport  VectorParamsAs1DForOutWhenUnconnected=off
  Q : Outport  Port=2  VectorParamsAs1DForOutWhenUnconnected=off
  wires:
  gain1/1 -> Q/1  "BESS Reactive Power(pu)"
  gain/1 -> P/1  "BESS Active Power(pu)"
  Low-Pass Filter (Discrete or Continuous)1/1 -> gain1/1
  Low-Pass Filter (Discrete or Continuous)/1 -> gain/1
  Vabc/1 -> Demux/1, Product/1
  Iabc/1 -> Product1/1, Product/2
  Product/1 -> Sum of Elements/1
  Sum of Elements/1 -> Low-Pass Filter (Discrete or Continuous)/1
  Demux/1 -> Minus2/2, Minus/1
  Demux/2 -> Minus1/1, Minus/2
  Demux/3 -> Minus2/1, Minus1/2
  Mux/1 -> Product1/2
  Product1/1 -> Sum of Elements1/1
  Sum of Elements1/1 -> Gain/1
  Gain/1 -> Low-Pass Filter (Discrete or Continuous)1/1
  Minus1/1 -> Mux/1
  Minus2/1 -> Mux/2
  Minus/1 -> Mux/3

== system IndustrialMicrogrid/MG1 Primary Substation/BESS and Controller/BESS/Grid-Forming Converter Control/Current Limiting/CurrentLimitingMethod/currentLimitAndVirtual/Current Saturation/Compare ==
  u : Inport
  Compare To Zero : simulink/Logic and Bit Operations/Compare To Zero  relop=<=  OutDataTypeStr=boolean
  Data Type Conversion : DataTypeConversion  SaturateOnIntegerOverflow=off  RndMeth=Floor
  Out1 : Outport
  wires:
  Compare To Zero/1 -> Data Type Conversion/1
  u/1 -> Compare To Zero/1
  Data Type Conversion/1 -> Out1/1

== system IndustrialMicrogrid/MG1 Primary Substation/BESS and Controller/BESS/Grid-Forming Converter Control/Current Limiting/CurrentLimitingMethod/currentLimitAndVirtual/Current Saturation/If Action Subsystem ==
  Is : Inport
  Isd : Inport  Port=2
  Isq : Inport  Port=3
  maxI : Inport  Port=4
  Action Port : ActionPort
  Divide : Product  Inputs=*/
  Product : Product
  Product1 : Product
  Idmax : Outport
  Iqmax : Outport  Port=2
  wires:
  maxI/1 -> Divide/1
  Is/1 -> Divide/2
  Divide/1 -> Product1/2, Product/1
  Isd/1 -> Product1/1
  Isq/1 -> Product/2
  Product1/1 -> Idmax/1
  Product/1 -> Iqmax/1

== system IndustrialMicrogrid/MG1 Primary Substation/BESS and Controller/BESS/Grid-Forming Converter Control/Current Limiting/CurrentLimitingMethod/currentLimitAndVirtual/Current Saturation/If Action Subsystem1 ==
  Action Port : ActionPort
  Constant3 : Constant  Value=0
  Constant4 : Constant  Value=0
  Idmax : Outport
  Iqmax : Outport  Port=2
  wires:
  Constant4/1 -> Iqmax/1
  Constant3/1 -> Idmax/1

== system IndustrialMicrogrid/MG1 Primary Substation/BESS and Controller/BESS/Grid-Forming Converter Control/Measurement/Frequency Measurement/Frequency Measurement/If Action Subsystem/Frequency estimation ==
  sk : Inport
  sk-1 : Inport  Port=2
  k : Inport  Port=3
  k-1 : Inport  Port=4
  Trigger : TriggerPort  VariantControl=(inherit)  InitialTriggerSignalState=positive
  Add1 : Sum  Inputs=+-  AccumDataTypeStr=double  OutDataTypeStr=double  RndMeth=Convergent
  Add2 : Sum
  Constant : Constant
  Delay : Delay  DelayLength=1
  Delay1 : Delay  DelayLength=1
  Divide : Product  Inputs=*/  RndMeth=Ceiling
  Gain : Gain  Gain=2  ParamDataTypeStr=double  RndMeth=Convergent
  Gain2 : Gain  Gain=0.5
  MATLAB Function : MATLAB Function  TreatAsAtomicUnit=on
  f : Outport
  wires:
  Add1/1 -> Gain/1
  Constant/1 -> Divide/1
  Gain/1 -> Divide/2
  MATLAB Function/1(x) -> Delay/1, Add1/1  "x1-y1/slope"
  Divide/1 -> Add2/1, Delay1/1
  Delay1/1 -> Add2/2
  Add2/1 -> Gain2/1
  Gain2/1 -> f/1
  Delay/1 -> Add1/2
  k/1 -> MATLAB Function/3(x1)
  k-1/1 -> MATLAB Function/4(x2)  "x1"
  sk/1 -> MATLAB Function/1(y1)
  sk-1/1 -> MATLAB Function/2(y2)

== system IndustrialMicrogrid/MG1 Primary Substation/BESS and Controller/BESS/Grid-Forming Converter Control/Power Control/ActivePowerControl/vsmControl/Damping Frequency/ConstantFreqReference ==
  fref : Inport
  Constant1 : Constant
  Terminator : Terminator
  fmeas : Outport
  wires:
  Constant1/1 -> fmeas/1
  fref/1 -> Terminator/1

== system IndustrialMicrogrid/MG1 Primary Substation/BESS and Controller/BESS/Grid-Forming Converter Control/Power Control/ActivePowerControl/vsmControl/Damping Frequency/WithFrequencyMeasurement ==
  fref : Inport
  fmeas : Outport
  wires:
  fref/1 -> fmeas/1

== system IndustrialMicrogrid/MG1 Primary Substation/BESS and Controller/BESS/Grid-Forming Converter Control/Power Control/ActivePowerControl/vsmControl/Power Reference Selection/If Action Subsystem ==
  note: Frequency difference power
  Pref : Inport
  Wsm : Inport  Port=2
  Action Port : ActionPort  ActionPortLabel=if(u1 > 0)
  Constant : Constant
  Gain6 : Gain  Gain=vsmFreqDroop
  Sum : Sum  Inputs=|+-
  Sum3 : Sum  Inputs=++|
  Power : Outport
  wires:
  Gain6/1 -> Sum3/2
  Pref/1 -> Sum3/1  "Reference power"
  Wsm/1 -> Sum/2
  Sum/1 -> Gain6/1
  Constant/1 -> Sum/1
  Sum3/1 -> Power/1

== system IndustrialMicrogrid/MG1 Primary Substation/BESS and Controller/BESS/Grid-Forming Converter Control/Power Control/ActivePowerControl/vsmControl/Power Reference Selection/If Action Subsystem1 ==
  note: Frequency difference power
  fref : Inport
  Wsm : Inport  Port=2
  Action Port : ActionPort  ActionPortLabel=else
  Gain6 : Gain  Gain=vsmFreqDroop
  Scope : Scope
  Scope1 : Scope
  Sum : Sum  Inputs=|+-
  Power : Outport
  wires:
  Wsm/1 -> Scope/1, Sum/2
  Sum/1 -> Gain6/1
  fref/1 -> Sum/1
  Gain6/1 -> Scope1/1, Power/1

== system IndustrialMicrogrid/MG2 Primary Substation/BESS and Controller 2/BESS/Grid-Forming Converter Control/Current Limiting/CurrentLimitingMethod/currentLimitAndVirtual/Current Saturation/Compare ==
  u : Inport
  Compare To Zero : simulink/Logic and Bit Operations/Compare To Zero  relop=<=  OutDataTypeStr=boolean
  Data Type Conversion : DataTypeConversion  SaturateOnIntegerOverflow=off  RndMeth=Floor
  Out1 : Outport
  wires:
  Compare To Zero/1 -> Data Type Conversion/1
  u/1 -> Compare To Zero/1
  Data Type Conversion/1 -> Out1/1

== system IndustrialMicrogrid/MG2 Primary Substation/BESS and Controller 2/BESS/Grid-Forming Converter Control/Current Limiting/CurrentLimitingMethod/currentLimitAndVirtual/Current Saturation/If Action Subsystem ==
  Is : Inport
  Isd : Inport  Port=2
  Isq : Inport  Port=3
  maxI : Inport  Port=4
  Action Port : ActionPort
  Divide : Product  Inputs=*/
  Product : Product
  Product1 : Product
  Idmax : Outport
  Iqmax : Outport  Port=2
  wires:
  maxI/1 -> Divide/1
  Is/1 -> Divide/2
  Divide/1 -> Product1/2, Product/1
  Isd/1 -> Product1/1
  Isq/1 -> Product/2
  Product1/1 -> Idmax/1
  Product/1 -> Iqmax/1

== system IndustrialMicrogrid/MG2 Primary Substation/BESS and Controller 2/BESS/Grid-Forming Converter Control/Current Limiting/CurrentLimitingMethod/currentLimitAndVirtual/Current Saturation/If Action Subsystem1 ==
  Action Port : ActionPort
  Constant3 : Constant  Value=0
  Constant4 : Constant  Value=0
  Idmax : Outport
  Iqmax : Outport  Port=2
  wires:
  Constant4/1 -> Iqmax/1
  Constant3/1 -> Idmax/1

== system IndustrialMicrogrid/MG2 Primary Substation/BESS and Controller 2/BESS/Grid-Forming Converter Control/Measurement/Frequency Measurement/Frequency Measurement/If Action Subsystem/Frequency estimation ==
  sk : Inport
  sk-1 : Inport  Port=2
  k : Inport  Port=3
  k-1 : Inport  Port=4
  Trigger : TriggerPort  VariantControl=(inherit)  InitialTriggerSignalState=positive
  Add1 : Sum  Inputs=+-  AccumDataTypeStr=double  OutDataTypeStr=double  RndMeth=Convergent
  Add2 : Sum
  Constant : Constant
  Delay : Delay  DelayLength=1
  Delay1 : Delay  DelayLength=1
  Divide : Product  Inputs=*/  RndMeth=Ceiling
  Gain : Gain  Gain=2  ParamDataTypeStr=double  RndMeth=Convergent
  Gain2 : Gain  Gain=0.5
  MATLAB Function : MATLAB Function  TreatAsAtomicUnit=on
  f : Outport
  wires:
  Add1/1 -> Gain/1
  Constant/1 -> Divide/1
  Gain/1 -> Divide/2
  MATLAB Function/1(x) -> Delay/1, Add1/1  "x1-y1/slope"
  Divide/1 -> Add2/1, Delay1/1
  Delay1/1 -> Add2/2
  Add2/1 -> Gain2/1
  Gain2/1 -> f/1
  Delay/1 -> Add1/2
  k/1 -> MATLAB Function/3(x1)
  k-1/1 -> MATLAB Function/4(x2)  "x1"
  sk/1 -> MATLAB Function/1(y1)
  sk-1/1 -> MATLAB Function/2(y2)

== system IndustrialMicrogrid/MG2 Primary Substation/BESS and Controller 2/BESS/Grid-Forming Converter Control/Power Control/ActivePowerControl/vsmControl/Damping Frequency/ConstantFreqReference ==
  fref : Inport
  Constant1 : Constant
  Terminator : Terminator
  fmeas : Outport
  wires:
  Constant1/1 -> fmeas/1
  fref/1 -> Terminator/1

== system IndustrialMicrogrid/MG2 Primary Substation/BESS and Controller 2/BESS/Grid-Forming Converter Control/Power Control/ActivePowerControl/vsmControl/Damping Frequency/WithFrequencyMeasurement ==
  fref : Inport
  fmeas : Outport
  wires:
  fref/1 -> fmeas/1

== system IndustrialMicrogrid/MG2 Primary Substation/BESS and Controller 2/BESS/Grid-Forming Converter Control/Power Control/ActivePowerControl/vsmControl/Power Reference Selection/If Action Subsystem ==
  note: Frequency difference power
  Pref : Inport
  Wsm : Inport  Port=2
  Action Port : ActionPort  ActionPortLabel=if(u1 > 0)
  Constant : Constant
  Gain6 : Gain  Gain=vsmFreqDroop
  Sum : Sum  Inputs=|+-
  Sum3 : Sum  Inputs=++|
  Power : Outport
  wires:
  Gain6/1 -> Sum3/2
  Pref/1 -> Sum3/1  "Reference power"
  Wsm/1 -> Sum/2
  Sum/1 -> Gain6/1
  Constant/1 -> Sum/1
  Sum3/1 -> Power/1

== system IndustrialMicrogrid/MG2 Primary Substation/BESS and Controller 2/BESS/Grid-Forming Converter Control/Power Control/ActivePowerControl/vsmControl/Power Reference Selection/If Action Subsystem1 ==
  note: Frequency difference power
  fref : Inport
  Wsm : Inport  Port=2
  Action Port : ActionPort  ActionPortLabel=else
  Gain6 : Gain  Gain=vsmFreqDroop
  Scope : Scope
  Scope1 : Scope
  Sum : Sum  Inputs=|+-
  Power : Outport
  wires:
  Wsm/1 -> Scope/1, Sum/2
  Sum/1 -> Gain6/1
  fref/1 -> Sum/1
  Gain6/1 -> Scope1/1, Power/1

== stateflow chart IndustrialMicrogrid/MG2 Primary Substation/BESS and Controller 2/BESS/Grid-Forming Converter Control/Current Limiting/CurrentLimitingMethod/currentLimitAndVirtual/CurrentLimitSelection ==
  state Mode1_VI_ON
    entry:
    noCurrentLimit  = 0;
    viCurrentLimit = 1;
    satCurrentLimit = 0;
    ismax= maxVICurrentLimit;
    exit:
    noCurrentLimit  = 0;
    viCurrentLimit = 1;
    satCurrentLimit = 0;
    ismax= maxVICurrentLimit;
  state Start_Mode
    entry:
    noCurrentLimit  = 1;
    viCurrentLimit = 0;
    satCurrentLimit = 0;
    ismax= maxSatCurrentLimit;
    exit:
    noCurrentLimit  = 1;
    viCurrentLimit = 0;
    satCurrentLimit = 0;
    ismax= maxSatCurrentLimit;
  state Mode2_CurrentSat_ON
    entry:
    noCurrentLimit  = 0;
    viCurrentLimit = 0;
    satCurrentLimit = 1;
    ismax= maxSatCurrentLimit;
    exit:
    noCurrentLimit  = 0;
    viCurrentLimit = 0;
    satCurrentLimit = 1;
    ismax= maxSatCurrentLimit;
  state Mode3_CurrentSat_ON
    entry:
    noCurrentLimit  = 0;
    viCurrentLimit = 0;
    satCurrentLimit = 1;
    ismax= 1.1*maxVICurrentLimit;
    exit:
    noCurrentLimit  = 0;
    viCurrentLimit = 0;
    satCurrentLimit = 1;
    ismax= 1.1*maxVICurrentLimit;
  Start_Mode -> Mode1_VI_ON : [Is>1]
  (junction 28) -> Mode1_VI_ON : after(currentControlTs*10, sec)[(Is<ismax) && (Is>1) ]
  Mode3_CurrentSat_ON -> (junction 28) [order 1]
  (default) -> Start_Mode
  Mode1_VI_ON -> Start_Mode [order 2] : [Is<1]
  Mode1_VI_ON -> Mode2_CurrentSat_ON [order 1] : after(0.5/powerFreq, sec)[(Is>=maxSatCurrentLimit)]
  (junction 26) -> Start_Mode
  Mode3_CurrentSat_ON -> Mode2_CurrentSat_ON [order 2] : after(0.5/powerFreq, sec)[(Is>ismax)]
  Mode2_CurrentSat_ON -> Mode3_CurrentSat_ON : after(currentSatTime, sec)[satCurrentLimit>0]
  Mode3_CurrentSat_ON -> (junction 26) [order 3] : [Is<1]
  data: Is input; ismax output; noCurrentLimit output; viCurrentLimit output; satCurrentLimit output; maxSatCurrentLimit parameter; maxVICurrentLimit parameter; currentControlTs parameter; currentSatTime parameter; powerFreq parameter

== matlab function IndustrialMicrogrid/MG2 Primary Substation/BESS and Controller 2/BESS/Grid-Forming Converter Control/Measurement/Frequency Measurement/Frequency Measurement/If Action Subsystem/Frequency estimation/MATLAB Function ==
  data: y1 input; y2 input; x1 input; x output; x2 input
function x = fcn(y1,y2,x1,x2)
% Line equation between two points is y-y1=((y2-y1)/(x2-x1))*(x-x1). Here
% to to find the zero crossing instant substitute y = 0 and find x
slope = (y2-y1)/(x2-x1);
x = x1-y1/slope;

== stateflow chart IndustrialMicrogrid/MG1 Primary Substation/BESS and Controller/BESS/Grid-Forming Converter Control/Current Limiting/CurrentLimitingMethod/currentLimitAndVirtual/CurrentLimitSelection ==
  state Mode1_VI_ON
    entry:
    noCurrentLimit  = 0;
    viCurrentLimit = 1;
    satCurrentLimit = 0;
    ismax= maxVICurrentLimit;
    exit:
    noCurrentLimit  = 0;
    viCurrentLimit = 1;
    satCurrentLimit = 0;
    ismax= maxVICurrentLimit;
  state Start_Mode
    entry:
    noCurrentLimit  = 1;
    viCurrentLimit = 0;
    satCurrentLimit = 0;
    ismax= maxSatCurrentLimit;
    exit:
    noCurrentLimit  = 1;
    viCurrentLimit = 0;
    satCurrentLimit = 0;
    ismax= maxSatCurrentLimit;
  state Mode2_CurrentSat_ON
    entry:
    noCurrentLimit  = 0;
    viCurrentLimit = 0;
    satCurrentLimit = 1;
    ismax= maxSatCurrentLimit;
    exit:
    noCurrentLimit  = 0;
    viCurrentLimit = 0;
    satCurrentLimit = 1;
    ismax= maxSatCurrentLimit;
  state Mode3_CurrentSat_ON
    entry:
    noCurrentLimit  = 0;
    viCurrentLimit = 0;
    satCurrentLimit = 1;
    ismax= 1.1*maxVICurrentLimit;
    exit:
    noCurrentLimit  = 0;
    viCurrentLimit = 0;
    satCurrentLimit = 1;
    ismax= 1.1*maxVICurrentLimit;
  Start_Mode -> Mode1_VI_ON : [Is>1]
  (junction 28) -> Mode1_VI_ON : after(currentControlTs*10, sec)[(Is<ismax) && (Is>1) ]
  Mode3_CurrentSat_ON -> (junction 28) [order 1]
  (default) -> Start_Mode
  Mode1_VI_ON -> Start_Mode [order 2] : [Is<1]
  Mode1_VI_ON -> Mode2_CurrentSat_ON [order 1] : after(0.5/powerFreq, sec)[(Is>=maxSatCurrentLimit)]
  (junction 26) -> Start_Mode
  Mode3_CurrentSat_ON -> Mode2_CurrentSat_ON [order 2] : after(0.5/powerFreq, sec)[(Is>ismax)]
  Mode2_CurrentSat_ON -> Mode3_CurrentSat_ON : after(currentSatTime, sec)[satCurrentLimit>0]
  Mode3_CurrentSat_ON -> (junction 26) [order 3] : [Is<1]
  data: Is input; ismax output; noCurrentLimit output; viCurrentLimit output; satCurrentLimit output; maxSatCurrentLimit parameter; maxVICurrentLimit parameter; currentControlTs parameter; currentSatTime parameter; powerFreq parameter
